simulink model "wind_loads"  (R2023a)
settings: Solver=ode4  StartTime=0.0  StopTime=10.0  FixedStep=0.01  RelTol=1e-3
values from neighbouring files (symbols this model uses):
  A_Fw = 2.9    [init_wind_loads.m]
  A_Lw = 8.6    [init_wind_loads.m]
  CD_lAF = 0.475    [init_wind_loads.m]
  CD_t = 0.9    [init_wind_loads.m]
  delta = 0.8    [init_wind_loads.m]
  H_Lw = 1.0    (= 1)    [init_wind_loads.m]
  kappa = 1.1    [init_wind_loads.m]
  L_oa = 5.0    (= 5)    [init_wind_loads.m]
  rho_air = 1.225    [init_wind_loads.m]
  s_L = 0.0    (= 0)    [init_wind_loads.m]
libraries: mssSimulink x2
settings Model: Creator=tobiasvt  LastModifiedBy=HalvorPlatou
settings SolverCC: AlgebraicLoopSolver=TrustRegion
settings DebuggingCC: UnconnectedInputMsg=warning  UnconnectedOutputMsg=warning  UnconnectedLineMsg=warning
settings ModelReferenceCC: EnableRefExpFcnMdlSchedulingChecks=on
settings RTWCC: Description=FMU based on GRT (Functional Mock-up Unit)  SystemTargetFile=grtfmi.tlc  GenerateMakefile=off  TemplateMakefile=none  RetainRTWFile=on
settings STFCustomTargetCC: ConcurrentExecutionCompliant=off  CombineOutputUpdateFcns=on  CodeInterfacePackaging=Reusable function  GRTInterface=off  GenerateAllocFcn=on  UseToolchainInfoCompliant=off  SystemTargetFile=grtfmi.tlc
settings GRTTargetCC: ParMdlRefBuildCompliant=off  CompOptLevelCompliant=off  ConcurrentExecutionCompliant=off  MatFileLogging=off  CodeInterfacePackaging=Reusable function  CPPClassGenCompliant=off  GenerateAllocFcn=on  UseToolchainInfoCompliant=off

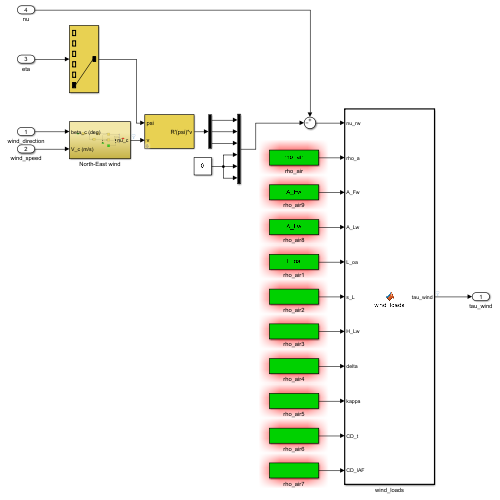
[thumbnail: Simulink's stored preview of the top-level diagram]
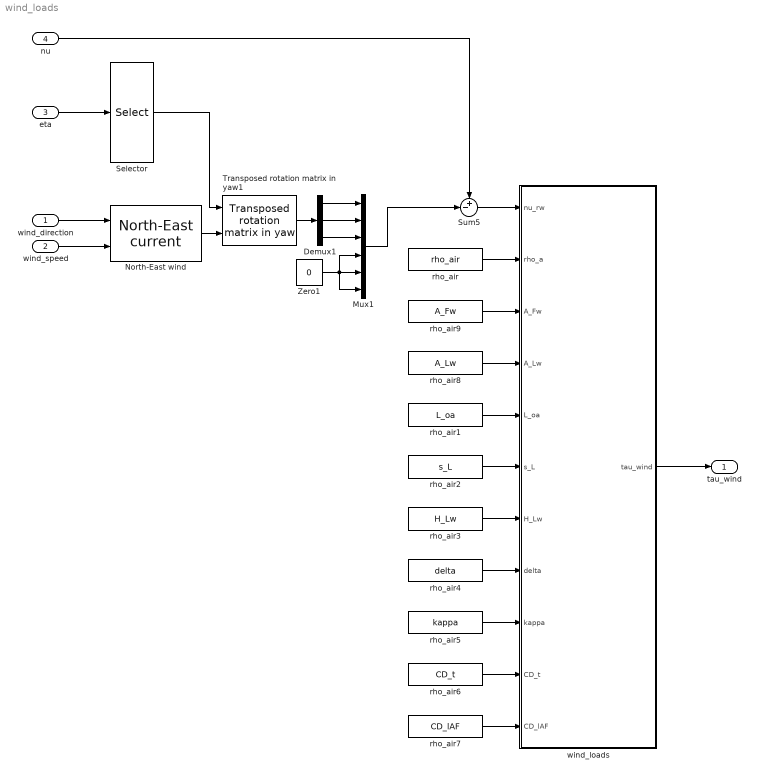
== system wind_loads ==
  wind_direction : Inport  PortDimensions=1
  wind_speed : Inport  Port=2  PortDimensions=1
  eta : Inport  Port=3  PortDimensions=6
  nu : Inport  Port=4  PortDimensions=6
  Demux1 : Demux  Outputs=3
  Mux1 : Mux  Inputs=6
  North-East wind : mssSimulink/Environment/Current/North-East current  SystemSampleTime=-1  VariantActivationTime=update diagram  Latency=0  AutoFrameSizeCalculation=off
  Selector : Selector  InputPortWidth=6  IndexOptions=Index vector (dialog)  Indices=[6]  OutputSizes=1
  Sum5 : Sum  Inputs=+-|
  Transposed rotation matrix in yaw1 : mssSimulink/Modelling/Kinematics/Transposed rotation  matrix in yaw
  Zero1 : Constant  Value=0  OutDataTypeStr=Inherit: Inherit via back propagation
  rho_air : Constant  Value=rho_air
  rho_air1 : Constant  Value=L_oa
  rho_air2 : Constant  Value=s_L
  rho_air3 : Constant  Value=H_Lw
  rho_air4 : Constant  Value=delta
  rho_air5 : Constant  Value=kappa
  rho_air6 : Constant  Value=CD_t
  rho_air7 : Constant  Value=CD_lAF
  rho_air8 : Constant  Value=A_Lw
  rho_air9 : Constant  Value=A_Fw
  wind_loads : MATLAB Function  TreatAsAtomicUnit=on
  tau_wind : Outport
  wires:
  Mux1/1 -> Sum5/2
  Transposed rotation matrix in yaw1/1 -> Demux1/1
  Demux1/2 -> Mux1/2
  Zero1/1 -> Mux1/6, Mux1/4, Mux1/5
  Demux1/1 -> Mux1/1
  wind_speed/1 -> North-East wind/2
  North-East wind/1 -> Transposed rotation matrix in yaw1/2
  Demux1/3 -> Mux1/3
  wind_direction/1 -> North-East wind/1
  Selector/1 -> Transposed rotation matrix in yaw1/1
  eta/1 -> Selector/1
  Sum5/1 -> wind_loads/1(nu_rw)
  nu/1 -> Sum5/1
  wind_loads/1(tau_wind) -> tau_wind/1
  rho_air/1 -> wind_loads/2(rho_a)
  rho_air9/1 -> wind_loads/3(A_Fw)
  rho_air8/1 -> wind_loads/4(A_Lw)
  rho_air1/1 -> wind_loads/5(L_oa)
  rho_air2/1 -> wind_loads/6(s_L)
  rho_air3/1 -> wind_loads/7(H_Lw)
  rho_air4/1 -> wind_loads/8(delta)
  rho_air5/1 -> wind_loads/9(kappa)
  rho_air6/1 -> wind_loads/10(CD_t)
  rho_air7/1 -> wind_loads/11(CD_lAF)

== matlab function wind_loads/wind_loads ==
  data: nu_rw input; rho_a input; tau_wind output; A_Fw input; A_Lw input; L_oa input; s_L input; H_Lw input; delta input; kappa input; CD_t input; CD_lAF input
function tau_wind = wind_loads(nu_rw, rho_a, A_Fw, A_Lw, L_oa, s_L, H_Lw, delta, kappa, CD_t, CD_lAF)
    gamma_rw = -atan2(nu_rw(2),nu_rw(1));
    V_rw = sqrt(nu_rw(1)^2 + nu_rw(2)^2);
    CD_l = CD_lAF*A_Fw/A_Lw;
    C_X = -CD_lAF*(cos(gamma_rw))/(1-0.5*delta*(1-(CD_l/CD_t))*sin(2*gamma_rw)^2);
    C_Y = CD_t*(sin(gamma_rw))/(1-0.5*delta*(1-(CD_l/CD_t))*sin(2*gamma_rw)^2);
    C_K = kappa*C_Y;
    C_N = ((s_L/L_oa) - 0.18*(abs(gamma_rw)-0.5*pi))*C_Y;
    
    tau_wind = 0.5*rho_a*V_rw^2*[C_X*A_Fw;
                                 C_Y*A_Lw;
                                 0.0;
                                 C_K*A_Lw*H_Lw;
                                 0.0;
                                 C_N*A_Lw*L_oa];
end
